simulink model "Commander_test"  (R2014b)
settings: Solver=ode3  StartTime=0.0  StopTime=60  RelTol=1e-3
libraries: BeagleBoneBlackCom x1
settings Model: SimulationMode=external  Creator=Sebastian  LastModifiedBy=Sebastian
settings OptimizationCC: OptimizeModelRefInitCode=on  LifeSpan=1  MaxStackSize=64
settings HardwareCC: ProdLargestAtomicInteger=Long  ProdLargestAtomicFloat=Double  ProdEndianess=LittleEndian  ProdHWDeviceType=ARM Compatible->ARM Cortex
settings RTWCC: SystemTargetFile=ert.tlc  TLCOptions=-aInlineSetEventsForThisBaseRateFcn=TLC_FALSE -aSuppressMultiTaskScheduler=TLC_FALSE  TemplateMakefile=ert_default_tmf  Description=Embedded Coder  GenerateReport=on  ProcessScript=ert_make_rtw_hook  Toolchain=Linaro Toolchain v4.8  BuildConfiguration=Specify  IncludeHyperlinkInReport=on  LaunchReport=on  GenerateTraceInfo=on  GenerateTraceReport=on  GenerateTraceReportSl=on  GenerateTraceReportSf=on  GenerateTraceReportEml=on
settings CodeAppCC: IgnoreCustomStorageClasses=off
settings ERTTargetCC: TargetLangStandard=C99 (ISO)  SupportNonInlinedSFcns=on  SupportVariableSizeSignals=on

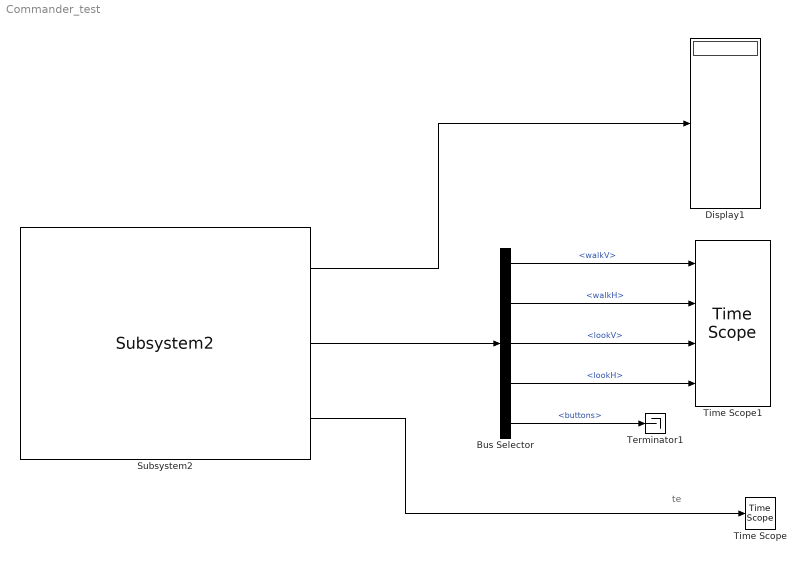
== system Commander_test ==
  note: te
  Bus Selector : BusSelector  OutputSignals=walkV,walkH,lookV,lookH,buttons
  Display1 : Display
  Subsystem2 : BeagleBoneBlackCom/Subsystem2  portNbr=Uart 2
  Terminator1 : Terminator
  Time Scope : TimeScope  DefaultConfigurationName=spbscopes.TimeScopeBlockCfg
  Time Scope1 : TimeScope  DefaultConfigurationName=spbscopes.TimeScopeBlockCfg  NumInputPorts=4
  wires:
  Subsystem2/1 -> Display1/1
  Subsystem2/3 -> Time Scope/1
  Subsystem2/2 -> Bus Selector/1
  Bus Selector/1 -> Time Scope1/1  "<walkV>"
  Bus Selector/2 -> Time Scope1/2  "<walkH>"
  Bus Selector/3 -> Time Scope1/3  "<lookV>"
  Bus Selector/4 -> Time Scope1/4  "<lookH>"
  Bus Selector/5 -> Terminator1/1  "<buttons>"
